simulink model "FastToSlow"  (Simulink 6.3)
settings: Solver=ode45  StartTime=0.0  StopTime=FastClk*300  RelTol=1e-3
PreLoadFcn:
  | disp('  > Setting clock period in Model pre-load function');
  | FastClk=1e-8
  | SlowClk=4e-8
InitFcn:
  | %% DSPBuilder Start
  | alt_dspbuilder_update_model(bdroot)
  | %% DSPBuilder End
libraries: allblocks_alteradspbuilder2 x16
settings Model: LastModifiedBy=LKONG  StrictBusMsg=None
settings DataIOCC: SignalLoggingName=sigsOut
settings OptimizationCC: InlineInvariantSignals=on
settings DebuggingCC: SolverPrmCheckMsg=none
settings HardwareCC: TargetUnknown=on

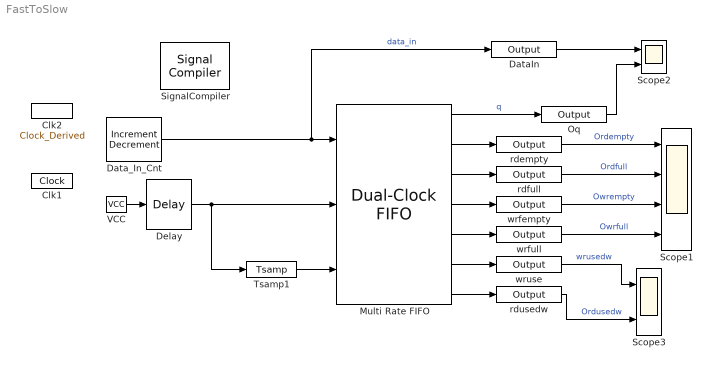
== system FastToSlow ==
  Clk1 : allblocks_alteradspbuilder2/Clock  ClockPeriod=40.0  ClockPeriodUnit=ns  SampleTime=4e-008  SimulationStartCycle=5  PhaseOffset=0  Reset=aclr  ResetType=Active Low  Export=off
  Clk2 : allblocks_alteradspbuilder2/Clock_Derived  ClockNumerator=1  ClockDenominator=4  SimulationStartCycle=5  PhaseOffset=0  Reset=aclr1  ResetType=Active Low  Export=off
  DataIn : allblocks_alteradspbuilder2/Output  iofile=d:\altera\70\dsPBuilder\DesignExamples\Tutorials\MultiRate\FIFO\tb_FastToSlow\FastToSlow_DataIn.capture  BusType=Signed Integer  bwl=8  bwr=0  PORTTYPE=Output
  Data_In_Cnt : allblocks_alteradspbuilder2/Increment Decrement  BusType=Signed Integer  bwl=8  bwr=0  SpecifyClock=on  clock=Clk2  clr_value=0  direction=Increment  phase_selection=1  use_ena=off  use_sclr=off
  Delay : allblocks_alteradspbuilder2/Delay  pipeline=3  ClockPhase=1  use_ena=off  use_sclr=off
  Multi Rate FIFO : allblocks_alteradspbuilder2/Dual-Clock FIFO  numwords=40  BusType=Signed Integer  bwl=8  bwr=0  ram_type=AUTO  UseBaseWriteClock=off  write_clock=Clk2  UseBaseReadClock=off  read_clock=Clk1  use_rdempty=on  use_rdfull=on  use_rdusedw=on  use_wrempty=on  use_wrfull=on  use_wrusedw=on  use_user_aclr=off  register_output=off  use_les_only=off  showahead_mode=off  synchronized=off
  Oq : allblocks_alteradspbuilder2/Output  iofile=d:\altera\70\dsPBuilder\DesignExamples\Tutorials\MultiRate\FIFO\tb_FastToSlow\FastToSlow_Oq.capture  BusType=Signed Integer  bwl=8  bwr=0  PORTTYPE=Output
  Scope1 : Scope  NumInputPorts=4
      settings: YMin=-5~-5~-5~-5  YMax=5~5~5~5
  Scope2 : Scope  NumInputPorts=2
      settings: YMin=-5~-5  YMax=5~5  SaveName=ScopeData2
  Scope3 : Scope  NumInputPorts=2
      settings: YMin=-5~-5  YMax=5~5
  SignalCompiler : allblocks_alteradspbuilder2/Signal Compiler  DeviceFamily=Stratix III  DeviceName=AUTO  EnableSignalTap=off  SignalTapDepth=128  UseBoardBlock=off  StpUseDefaultClock=on  StpClock=clock
  Tsamp1 : allblocks_alteradspbuilder2/Tsamp  SpecifyClock=on  clock=Clk1
  VCC : allblocks_alteradspbuilder2/VCC  SpecifyClock=on  clock=Clk2
  rdempty : allblocks_alteradspbuilder2/Output  iofile=d:\altera\70\dsPBuilder\DesignExamples\Tutorials\MultiRate\FIFO\tb_FastToSlow\FastToSlow_rdempty.capture  BusType=Single Bit  bwl=1  bwr=0  PORTTYPE=Output
  rdfull : allblocks_alteradspbuilder2/Output  iofile=d:\altera\70\dsPBuilder\DesignExamples\Tutorials\MultiRate\FIFO\tb_FastToSlow\FastToSlow_rdfull.capture  BusType=Single Bit  bwl=1  bwr=0  PORTTYPE=Output
  rdusedw : allblocks_alteradspbuilder2/Output  iofile=d:\altera\70\dsPBuilder\DesignExamples\Tutorials\MultiRate\FIFO\tb_FastToSlow\FastToSlow_rdusedw.capture  BusType=Signed Integer  bwl=8  bwr=0  PORTTYPE=Output
  wrfempty : allblocks_alteradspbuilder2/Output  iofile=d:\altera\70\dsPBuilder\DesignExamples\Tutorials\MultiRate\FIFO\tb_FastToSlow\FastToSlow_wrfempty.capture  BusType=Single Bit  bwl=1  bwr=0  PORTTYPE=Output
  wrfull : allblocks_alteradspbuilder2/Output  iofile=d:\altera\70\dsPBuilder\DesignExamples\Tutorials\MultiRate\FIFO\tb_FastToSlow\FastToSlow_wrfull.capture  BusType=Single Bit  bwl=1  bwr=0  PORTTYPE=Output
  wruse : allblocks_alteradspbuilder2/Output  iofile=d:\altera\70\dsPBuilder\DesignExamples\Tutorials\MultiRate\FIFO\tb_FastToSlow\FastToSlow_wruse.capture  BusType=Signed Integer  bwl=8  bwr=0  PORTTYPE=Output
  wires:
  Data_In_Cnt/1 -> Multi Rate FIFO/1, DataIn/1  "data_in"
  Multi Rate FIFO/4 -> wrfempty/1
  Multi Rate FIFO/5 -> wrfull/1
  Multi Rate FIFO/6 -> wruse/1
  VCC/1 -> Delay/1
  Multi Rate FIFO/7 -> rdusedw/1
  Multi Rate FIFO/1 -> Oq/1  "q"
  Multi Rate FIFO/2 -> rdempty/1
  Multi Rate FIFO/3 -> rdfull/1
  Delay/1 -> Tsamp1/1, Multi Rate FIFO/2
  Tsamp1/1 -> Multi Rate FIFO/3
  rdempty/1 -> Scope1/1  "Ordempty"
  rdfull/1 -> Scope1/2  "Ordfull"
  wrfempty/1 -> Scope1/3  "Owrempty"
  wrfull/1 -> Scope1/4  "Owrfull"
  wruse/1 -> Scope3/1  "wrusedw"
  rdusedw/1 -> Scope3/2  "Ordusedw"
  Oq/1 -> Scope2/2
  DataIn/1 -> Scope2/1
